simulink model "Lab03"  (Simulink 7.4)
settings: Solver=ode45  StartTime=0.0  StopTime=10.0  RelTol=1e-3
libraries: cstblocks x3
settings Model: Creator=AshfaqAhmad  LastModifiedBy=AshfaqAhmad

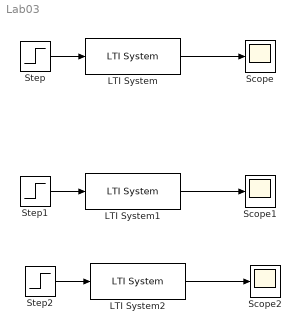
== system Lab03 ==
  LTI System : cstblocks/LTI System  SystemSampleTime=-1  sys=tf(30,[1 5 10])  IC=[]
  LTI System1 : cstblocks/LTI System  SystemSampleTime=-1  sys=tf(30,[1 0 10])  IC=[]
  LTI System2 : cstblocks/LTI System  SystemSampleTime=-1  sys=tf(30,[3 -2 10])  IC=[]
  Scope : Scope
  Scope1 : Scope
  Scope2 : Scope
      settings: SaveName=ScopeData2
  Step : Step  SampleTime=0
  Step1 : Step  SampleTime=0
  Step2 : Step  SampleTime=0
  wires:
  LTI System/1 -> Scope/1
  Step/1 -> LTI System/1
  LTI System1/1 -> Scope1/1
  Step1/1 -> LTI System1/1
  LTI System2/1 -> Scope2/1
  Step2/1 -> LTI System2/1
